simulink model "untitled11"  (R2024a)
settings: Solver=FixedStepAuto  StartTime=0.0  StopTime=10.0  RelTol=1e-3
libraries: androiduilib x3, androidaudiovideolib x1, androidcommunicationlib x1
settings Model: Creator=bhand  LastModifiedBy=Prashant Mahawar
settings OptimizationCC: DefaultParameterBehavior=Inlined  EnhancedBackFolding=on  PassReuseOutputArgsAs=Individual arguments  ZeroExternalMemoryAtStartup=off  ZeroInternalMemoryAtStartup=off  MaxStackSize=64  OptimizeBlockOrder=speed  DifferentSizesBufferReuse=on  OptimizationCustomize=off  EfficientTunableParamExpr=on
settings DebuggingCC: ParameterTunabilityLossMsg=error
settings HardwareCC: ProdBitPerLong=64  ProdLargestAtomicInteger=LongLong  ProdLargestAtomicFloat=Double  ProdLongLongMode=on  ProdHWDeviceType=ARM Compatible->ARM Cortex-A (64-bit)  UseEmbeddedCoderFeatures=off  UseSimulinkCoderFeatures=off
settings SFSimCC: MATLABDynamicMemAlloc=off
settings RTWCC: Description=Embedded Coder  SystemTargetFile=ert.tlc  HardwareBoard=Android Device (64bit)  TLCOptions="-aInlineSetEventsForThisBaseRateFcn=TLC_FALSE -aSuppressMultiTaskScheduler=TLC_FALSE  -aRateBasedStepFcn=0"  TemplateMakefile=ert_default_tmf  RTWVerbose=off  Toolchain=Android SDK/NDK Tools
settings CodeAppCC: ForceParamTrailComments=on  IgnoreCustomStorageClasses=off  OperatorAnnotations=on  SimulinkDataObjDesc=on  SFDataObjDesc=on  InsertBlockDesc=on
settings ERTTargetCC: SupportNonInlinedSFcns=on  InlinedParameterPlacement=NonHierarchical

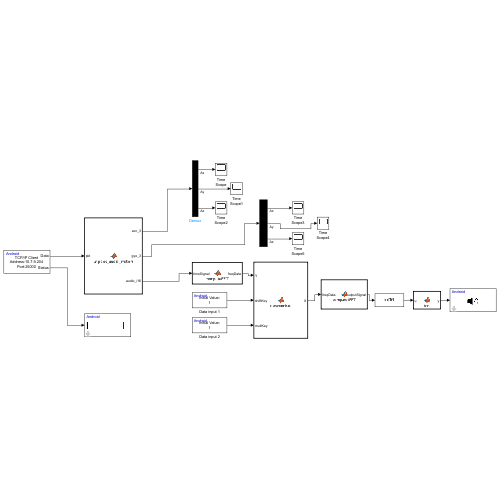
[thumbnail: Simulink's stored preview of the top-level diagram]
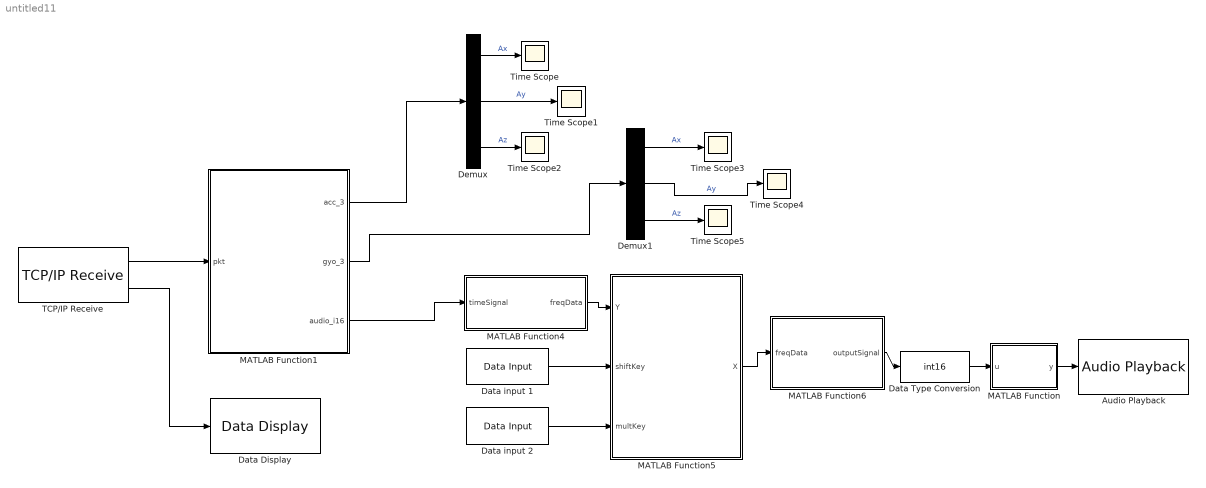
== system untitled11 ==
  Audio Playback : androidaudiovideolib/Audio Playback  SampleFreq=44100  AudioSamplingFreq=44100  SampleTime=0.1  DeviceStr=0  QueueDuration=0  BlockPlatform=Android
  Data Display : androiduilib/Data Display  DataDisplayId=untitled11/Data_Display  Format=Float  Precision=6  SimulateUsing=Code generation  blockPlatform=Android
  Data Type Conversion : DataTypeConversion  OutDataTypeStr=int16  SaturateOnIntegerOverflow=off  RndMeth=Floor
  Data input 1 : androiduilib/Data Input  isCharVector=off  Value=1.0  CharVector=Hello World  OutputDataType=int8  maxCharVectorSize=100  DataInputId=untitled11/Key_1  SampleTime=0.1
  Data input 2 : androiduilib/Data Input  isCharVector=off  Value=1.0  CharVector=Hello World  OutputDataType=int8  maxCharVectorSize=100  DataInputId=untitled11/Key_1  SampleTime=0.1
  Demux : Demux  Outputs=3
  Demux1 : Demux  Outputs=3
  MATLAB Function : MATLAB Function  TreatAsAtomicUnit=on
  MATLAB Function1 : MATLAB Function  TreatAsAtomicUnit=on
  MATLAB Function4 : MATLAB Function  TreatAsAtomicUnit=on
  MATLAB Function5 : MATLAB Function  TreatAsAtomicUnit=on
  MATLAB Function6 : MATLAB Function  TreatAsAtomicUnit=on
  TCP/IP Receive : androidcommunicationlib/TCP//IP Receive  TCPReceiveId=untitled11/TCP//IP_Receive  Mode_=Client  LocalServerPort_=25000  RemoteAddr_=10.7.9.204  RemoteServerPort_=25000  DataType_=uint8  DataSize_=8848  SampleTime_=0.1  ClientPortBindingSelection_=off  ClientPortToBind_=35000  BlockingMode_=off  BlockTimeout_=0.1
  Time Scope{,1..5} (6 alike) : Scope
  wires:
  MATLAB Function/1(y) -> Audio Playback/1
  Data Type Conversion/1 -> MATLAB Function/1(u)
  MATLAB Function6/1(outputSignal) -> Data Type Conversion/1
  MATLAB Function4/1(freqData) -> MATLAB Function5/1(Y)
  MATLAB Function1/3(audio_i16) -> MATLAB Function4/1(timeSignal)
  MATLAB Function5/1(X) -> MATLAB Function6/1(freqData)
  Data input 1/1 -> MATLAB Function5/2(shiftKey)
  MATLAB Function1/1(acc_3) -> Demux/1
  TCP/IP Receive/1 -> MATLAB Function1/1(pkt)
  TCP/IP Receive/2 -> Data Display/1
  Data input 2/1 -> MATLAB Function5/3(multKey)
  MATLAB Function1/2(gyo_3) -> Demux1/1
  Demux1/1 -> Time Scope3/1  "Ax"
  Demux1/2 -> Time Scope4/1  "Ay"
  Demux1/3 -> Time Scope5/1  "Az"
  Demux/1 -> Time Scope/1  "Ax"
  Demux/2 -> Time Scope1/1  "Ay"
  Demux/3 -> Time Scope2/1  "Az"

== matlab function untitled11/MATLAB Function1 ==
  data: pkt input; acc_3 output size=6; gyo_3 output; audio_i16 output size=4410
function [acc_3,gyo_3, audio_i16] = unpack_audio_motion(pkt)
%Extracting only the motion and audio values as sync was there in pack fnc
    acc_3   = typecast(pkt(5:16), 'single');
    gyo_3   = typecast(pkt(17:28), 'single');
    audio_i16 = typecast(pkt(29:8848), 'int16');
end

== matlab function untitled11/MATLAB Function ==
  data: u input; y output
function y = fcn(u)
% Converting int16 audio stream to int16 [N x 2] output for Android speaker

% Ensuring column vector
u = u(:);

% Normalizing to [-1, 1] in double
x = double(u) / double(intmax('int16'));

% Scaling back to int16
x_int16 = int16(x * double(intmax('int16')));

% Duplicating into two channels [N x 2]
y = [x_int16, x_int16];

end

== matlab function untitled11/MATLAB Function4 ==
  data: timeSignal input; freqData output
function freqData = computeFFT(timeSignal)

% Verify input is a vector
assert(isvector(timeSignal), 'computeFFT: timeSignal must be a vector.');

% Track input orientation (row or column)
inputWasRow = isrow(timeSignal);

% Convert input to single precision column vector
timeSignal = single(timeSignal(:));
numSamples = length(timeSignal);

% Perform FFT and normalize to prevent amplitude scaling
freqData = fft(timeSignal) / single(numSamples);

% Preserve the input shape
if inputWasRow
    freqData = freqData.';
end
end

== matlab function untitled11/MATLAB Function5 ==
  data: Y input; X output; shiftKey input; multKey input
function X = descramble(Y, shiftKey, multKey)
%#codegen
% descramble - Reverses the scrambling operation.
%
% Inputs:
%   Y         : Scrambled frequency-domain input (vector)
%   shiftKey  : Number of bins originally right-shifted
%   multKey   : Magnitude multiplier used during scrambling
%
% Output:
%   X         : Recovered (descrambled) frequency-domain data

% Ensure input is a vector
assert(isvector(Y), 'Input must be a vector.');

% Make sure keys are numeric
shiftKey = double(shiftKey);
multKey  = double(multKey);

% Step 1: Undo magnitude scaling
X = abs(Y) / multKey .* exp(1j * angle(Y));

% Step 2: Undo the circular shift (left shift)
X = circshift(X, -shiftKey);

end

== matlab function untitled11/MATLAB Function6 ==
  data: freqData input; outputSignal output
function outputSignal = computeIFFT(freqData)

% Ensure input is a vector
assert(isvector(freqData), 'computeIFFT: freqData must be a vector.');

% Check orientation (row or column)
inputWasRow = isrow(freqData);

% Convert input to a complex single-precision column vector
freqData = complex(single(freqData(:)));
numPts = length(freqData);

% Perform IFFT (multiply by N to undo FFT normalization)
tempResult = ifft(freqData * single(numPts));

% Extract the real part of the signal
outputSignal = real(tempResult);

% Preserve original shape
if inputWasRow
    outputSignal = outputSignal.';
end
end
